simulink model "sin_controlador"  (R2018b)
settings: Solver=VariableStepAuto  StartTime=0.0  StopTime=10.0  RelTol=1e-3
settings Model: Creator=root  LastModifiedBy=root

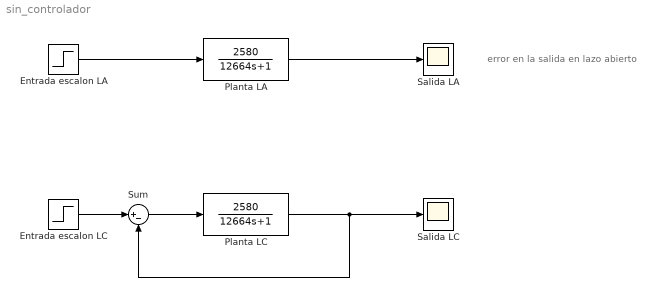
== system sin_controlador ==
  note: error en la salida en lazo abierto
  Entrada escalon LA : Step  Time=0  SampleTime=0
  Entrada escalon LC : Step  Time=0  SampleTime=0
  Planta LA : TransferFcn  Numerator=[2580]  Denominator=[12664 1]
  Planta LC : TransferFcn  Numerator=[2580]  Denominator=[12664 1]
  Salida LA : Scope
  Salida LC : Scope
  Sum : Sum  Inputs=|+-
  wires:
  Planta LC/1 -> Sum/2, Salida LC/1
  Entrada escalon LC/1 -> Sum/1
  Sum/1 -> Planta LC/1
  Entrada escalon LA/1 -> Planta LA/1
  Planta LA/1 -> Salida LA/1
